simulink model "KAL_PID"  (R2019a)
settings: Solver=FixedStepAuto  StartTime=0.0  StopTime=4/speed  FixedStep=0.005  MaxStep=1e-2  MinStep=1e-3  RelTol=5e-3
PreLoadFcn:
  | helperSLCreateUtilityBus;
  | createCostmap;
StopFcn:
  | clear helperSLVisualizePath;
values from neighbouring files (symbols this model uses):
  costmap = vehicleCostmap(circuit, 'cellSize', res )    [createCostmap.m]    (also in helperSLVisualizePath.m = vehicleCostmap(costmapStruct.Costs,          'FreeThreshold')
  curvatures = zeros(561,1)    [createCostmap.m]
  refPoses = zeros(561, 3)    [createCostmap.m]
  speed = 0.1    [createCostmap.m]
  startPose = refPoses(1,:)    [createCostmap.m]
libraries: simulink_extras x3, simulink x2, autolibshared x1
settings Model: Creator=The MathWorks, Inc.  LastModifiedBy=mingz
settings SolverCC: ZeroCrossAlgorithm=Adaptive  DecoupledContinuousIntegration=on  MinimalZcImpactIntegration=on
settings DataIOCC: SaveFormat=Array  SaveOutput=off  SignalLogging=off  DSMLogging=off  SaveTime=off  ReturnWorkspaceOutputs=off
settings OptimizationCC: UseDivisionForNetSlopeComputation=on
settings DebuggingCC: PregeneratedLibrarySubsystemCodeDiagnostic=none  ArithmeticOperatorsInVariantConditions=warning
settings SFSimCC: SimUseLocalCustomCode=off
settings RTWCC: RTWUseLocalCustomCode=off

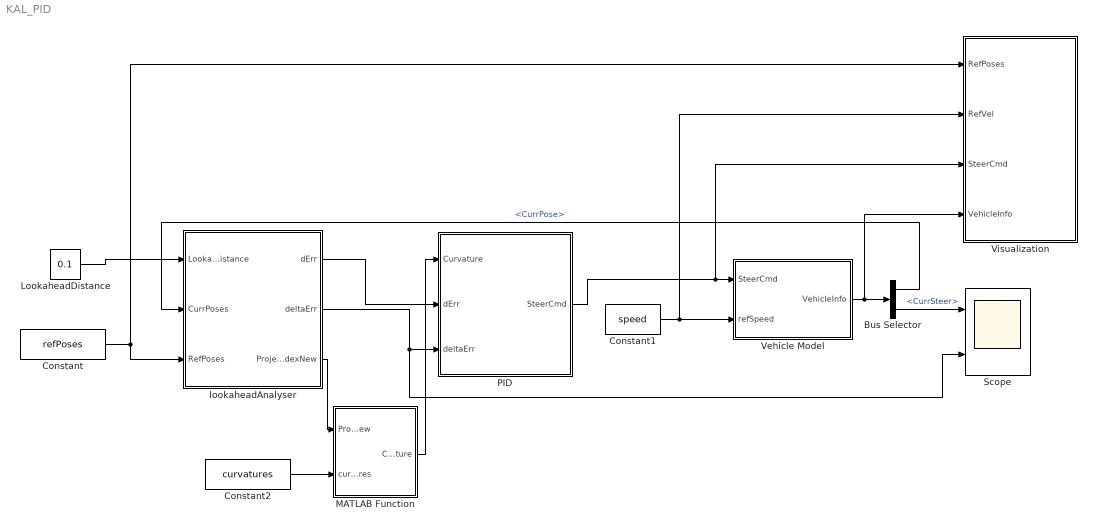
== system KAL_PID ==
  Bus Selector : BusSelector  OutputSignals=CurrPose,CurrSteer
  Constant : Constant  Value=refPoses
  Constant1 : Constant  Value=speed
  Constant2 : Constant  Value=curvatures
  LookaheadDistance : Constant  Value=0.1
  MATLAB Function : MATLAB Function  TreatAsAtomicUnit=on
  PID : Subsystem
  Scope : Scope  NumInputPorts=2
  Vehicle Model : Subsystem
  Visualization : Subsystem  mask{Costmap=costmap}
      mask prompts: Costmap "Vehicle costmap:"
      mask init:
      | validateattributes(Costmap, {'vehicleCostmap'}, {'scalar'});
      | 
      | varagout          = helperSLCreateUtilityStruct(Costmap);
      | vehicleDimsStruct = varagout{1};
      | costmapStruct     = varagout{2};
      mask DialogControl DescTextVar Prompt: Visualize simulation results.
  lookaheadAnalyser : Subsystem
  wires:
  Constant/1 -> Visualization/1(RefPoses), lookaheadAnalyser/3(RefPoses)
  Bus Selector/1 -> lookaheadAnalyser/2(CurrPoses)  "<CurrPose>"
  Bus Selector/2 -> Scope/1  "<CurrSteer>"
  Vehicle Model/1(VehicleInfo) -> Visualization/4(VehicleInfo), Bus Selector/1
  Constant1/1 -> Visualization/2(RefVel), Vehicle Model/2(refSpeed)
  lookaheadAnalyser/2(deltaErr) -> Scope/2, PID/3(deltaErr)
  lookaheadAnalyser/1(dErr) -> PID/2(dErr)
  lookaheadAnalyser/3(ProjectionLineIndexNew) -> MATLAB Function/1(ProjectionLineIndexNew)
  Constant2/1 -> MATLAB Function/2(curvatures)
  MATLAB Function/1(Curvature) -> PID/1(Curvature)
  PID/1(SteerCmd) -> Visualization/3(SteerCmd), Vehicle Model/1(SteerCmd)
  LookaheadDistance/1 -> lookaheadAnalyser/1(LookaheadDistance)

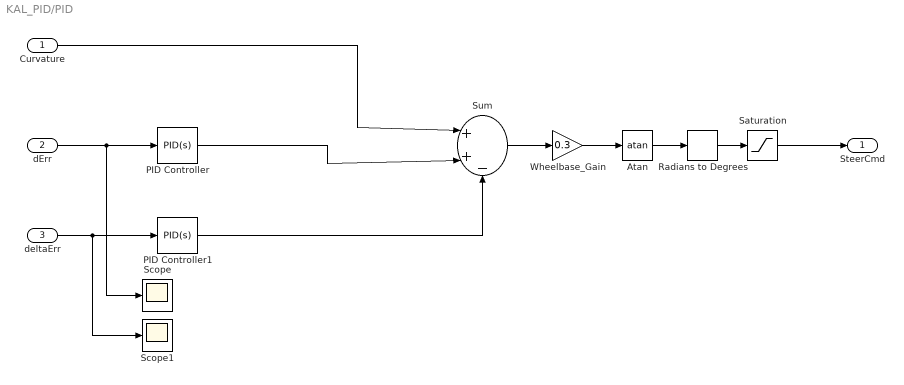
== system KAL_PID/PID ==
  Curvature : Inport
  dErr : Inport  Port=2
  deltaErr : Inport  Port=3
  Atan : Trigonometry  Operator=atan
  PID Controller : simulink/Continuous/PID Controller  Controller=PID  Form=Parallel  TimeDomain=Continuous-time  SampleTime=-1  IntegratorMethod=Forward Euler  FilterMethod=Forward Euler  ControllerParametersSource=internal  P=1  I=0  D=0.8  UseFilter=on  N=100  TunerSelectOption=Transfer Function Based (PID Tuner App)  InitialConditionSource=internal  InitialConditionForIntegrator=0  InitialConditionForFilter=0  DifferentiatorICPrevScaledInput=0  ExternalReset=none  TrackingMode=off  Kt=1  LimitOutput=off  UpperSaturationLimit=inf  LowerSaturationLimit=-inf  LinearizeAsGain=on  AntiWindupMode=none  Kb=1  POutMin=[]  POutMax=[]  IOutMin=[]  IOutMax=[]  DOutMin=[]  DOutMax=[]  NOutMin=[]  NOutMax=[]  SumOutMin=[]  SumOutMax=[]  SaturationOutMin=[]  SaturationOutMax=[]  PParamMin=[]  PParamMax=[]  IParamMin=[]  IParamMax=[]  DParamMin=[]  DParamMax=[]  NParamMin=[]  NParamMax=[]  KbParamMin=[]  KbParamMax=[]  KtParamMin=[]  KtParamMax=[]  KbOutMin=[]  KbOutMax=[]  KtOutMin=[]  KtOutMax=[]  IntegratorOutMin=[]  IntegratorOutMax=[]  FilterOutMin=[]  FilterOutMax=[]  SumI1OutMin=[]  SumI1OutMax=[]  SumI2OutMin=[]  SumI2OutMax=[]  SumI3OutMin=[]  SumI3OutMax=[]  SumI4OutMin=[]  SumI4OutMax=[]  SumDOutMin=[]  SumDOutMax=[]  DifferentiatorOutMin=[]  DifferentiatorOutMax=[]  FilterDiffOutCoefMin=[]  FilterDiffOutCoefMax=[]  ReciprocalOutMin=[]  ReciprocalOutMax=[]  SumDenOutMin=[]  SumDenOutMax=[]  SumNumOutMin=[]  SumNumOutMax=[]  DivideOutMin=[]  DivideOutMax=[]  IntegratorContinuousStateAttributes=''  IntegratorStateMustResolveToSignalObject=off  IntegratorRTWStateStorageClass=Auto  FilterContinuousStateAttributes=''  FilterStateMustResolveToSignalObject=off  FilterRTWStateStorageClass=Auto  ParallelPVariant=InternalParameters  IdealPVariant=Disabled  IVariant=InternalParameters  DVariant=InternalParameters  IntegratorVariant=Continuous  SatVariant=Disabled  AWVariant=Passthrough  PCopyVariant=Disabled  TRVariant=Disabled  FdbkBlocksVariant=Forward  IdealPFdbkVariant=Disabled  SatFdbkVariant=Disabled  DerivativeFilterVariant=ContFilter  NVariant=InternalParameters  NCopyVariant=Disabled  FilterICVariant=InternalICsFilter  IntegratorICVariant=InternalICs  ExternalResetVariant=Disabled  TRSumVariant=Passthrough  SumFdbkVariant=Disabled  SumVariant=Sum_PID
  PID Controller1 : simulink/Continuous/PID Controller  Controller=PID  Form=Parallel  TimeDomain=Continuous-time  SampleTime=-1  IntegratorMethod=Forward Euler  FilterMethod=Forward Euler  ControllerParametersSource=internal  P=2  I=0  D=0.6  UseFilter=on  N=100  TunerSelectOption=Transfer Function Based (PID Tuner App)  InitialConditionSource=internal  InitialConditionForIntegrator=0  InitialConditionForFilter=0  DifferentiatorICPrevScaledInput=0  ExternalReset=none  TrackingMode=off  Kt=1  LimitOutput=off  UpperSaturationLimit=inf  LowerSaturationLimit=-inf  LinearizeAsGain=on  AntiWindupMode=none  Kb=1  POutMin=[]  POutMax=[]  IOutMin=[]  IOutMax=[]  DOutMin=[]  DOutMax=[]  NOutMin=[]  NOutMax=[]  SumOutMin=[]  SumOutMax=[]  SaturationOutMin=[]  SaturationOutMax=[]  PParamMin=[]  PParamMax=[]  IParamMin=[]  IParamMax=[]  DParamMin=[]  DParamMax=[]  NParamMin=[]  NParamMax=[]  KbParamMin=[]  KbParamMax=[]  KtParamMin=[]  KtParamMax=[]  KbOutMin=[]  KbOutMax=[]  KtOutMin=[]  KtOutMax=[]  IntegratorOutMin=[]  IntegratorOutMax=[]  FilterOutMin=[]  FilterOutMax=[]  SumI1OutMin=[]  SumI1OutMax=[]  SumI2OutMin=[]  SumI2OutMax=[]  SumI3OutMin=[]  SumI3OutMax=[]  SumI4OutMin=[]  SumI4OutMax=[]  SumDOutMin=[]  SumDOutMax=[]  DifferentiatorOutMin=[]  DifferentiatorOutMax=[]  FilterDiffOutCoefMin=[]  FilterDiffOutCoefMax=[]  ReciprocalOutMin=[]  ReciprocalOutMax=[]  SumDenOutMin=[]  SumDenOutMax=[]  SumNumOutMin=[]  SumNumOutMax=[]  DivideOutMin=[]  DivideOutMax=[]  IntegratorContinuousStateAttributes=''  IntegratorStateMustResolveToSignalObject=off  IntegratorRTWStateStorageClass=Auto  FilterContinuousStateAttributes=''  FilterStateMustResolveToSignalObject=off  FilterRTWStateStorageClass=Auto  ParallelPVariant=InternalParameters  IdealPVariant=Disabled  IVariant=InternalParameters  DVariant=InternalParameters  IntegratorVariant=Continuous  SatVariant=Disabled  AWVariant=Passthrough  PCopyVariant=Disabled  TRVariant=Disabled  FdbkBlocksVariant=Forward  IdealPFdbkVariant=Disabled  SatFdbkVariant=Disabled  DerivativeFilterVariant=ContFilter  NVariant=InternalParameters  NCopyVariant=Disabled  FilterICVariant=InternalICsFilter  IntegratorICVariant=InternalICs  ExternalResetVariant=Disabled  TRSumVariant=Passthrough  SumFdbkVariant=Disabled  SumVariant=Sum_PID
  Radians to Degrees : simulink_extras/Transformations/Radians to Degrees
  Saturation : Saturate  UpperLimit=50  LowerLimit=-50
  Scope : Scope
  Scope1 : Scope
  Sum : Sum  Inputs=|++-
  Wheelbase_Gain : Gain  Gain=0.3
  SteerCmd : Outport
  wires:
  dErr/1 -> Scope/1, PID Controller/1
  PID Controller1/1 -> Sum/3
  Curvature/1 -> Sum/1
  Saturation/1 -> SteerCmd/1
  PID Controller/1 -> Sum/2
  Sum/1 -> Wheelbase_Gain/1
  Wheelbase_Gain/1 -> Atan/1
  Atan/1 -> Radians to Degrees/1
  Radians to Degrees/1 -> Saturation/1
  deltaErr/1 -> Scope1/1, PID Controller1/1

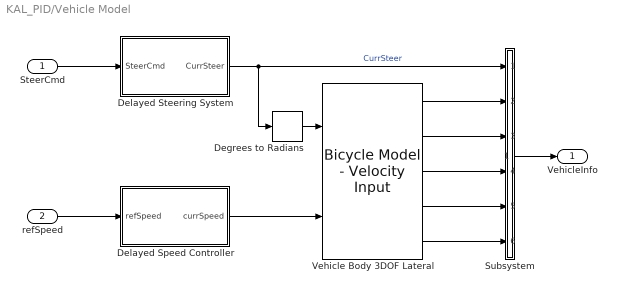
== system KAL_PID/Vehicle Model ==
  SteerCmd : Inport
  refSpeed : Inport  Port=2
  Degrees to Radians : simulink_extras/Transformations/Degrees to Radians
  Delayed Speed Controller : Subsystem
  Delayed Steering System : Subsystem
  Subsystem : Subsystem
  Vehicle Body 3DOF Lateral : autolibshared/Bicycle Model - Velocity Input  trackMode=Single (bicycle)  inputMode=External longitudinal forces  frontSteerMode=on  rearSteerMode=off  windMode=off  muMode=off  extFMode=off  extMMode=off  aMode=3  NF=2  NR=2  m=1.2  a=0.10  b=0.05  h=0.04  X_o=startPose(1)+cosd(startPose(3))*0.05  xdot_o=0  CalphaMode=off  sigmaMode=on  w=[1.4,1.4]  Cy_f=19e3  Cy_r=20e3  sigma_f=.1  sigma_r=.1  alpha_f_brk=[-.1 .1]  Cy_f_data=[-9e3 9e3]  alpha_r_brk=[-.1 .1]  Cy_r_data=[-9e3 9e3]  Y_o=startPose(2)+sind(startPose(3))*0.05  ydot_o=0  Izz=0.004  psi_o=deg2rad(startPose(3))  r_o=0  Af=2  Cd=.3  Cl=.1  Cpm=.1  beta_w=[0:0.01:0.3]  Cs=[0:0.03:0.9]  Cym=[0:0.01:0.3]  Pabs=101325  Tair=273  g=9.81  mu=1  xdot_tol=0.01  Fznom=5000  Fxtire_sat=1e6  Fytire_sat=1e6  longOff=0  latOff=0  vertOff=0
      settings: SourceProductName=Powertrain Blockset  SourceProductBaseCode=PW
  VehicleInfo : Outport
  wires:
  Delayed Speed Controller/1(currSpeed) -> Vehicle Body 3DOF Lateral/2
  Degrees to Radians/1 -> Vehicle Body 3DOF Lateral/1
  Delayed Steering System/1(CurrSteer) -> Degrees to Radians/1, Subsystem/1(CurrSteer)  "CurrSteer"
  SteerCmd/1 -> Delayed Steering System/1(SteerCmd)
  Subsystem/1(VehicleInfo) -> VehicleInfo/1
  Vehicle Body 3DOF Lateral/1 -> Subsystem/2(Info)
  Vehicle Body 3DOF Lateral/2 -> Subsystem/3(In3)
  Vehicle Body 3DOF Lateral/3 -> Subsystem/4(In4)
  Vehicle Body 3DOF Lateral/4 -> Subsystem/5(In6)
  Vehicle Body 3DOF Lateral/5 -> Subsystem/6(<Direction>)
  refSpeed/1 -> Delayed Speed Controller/1(refSpeed)

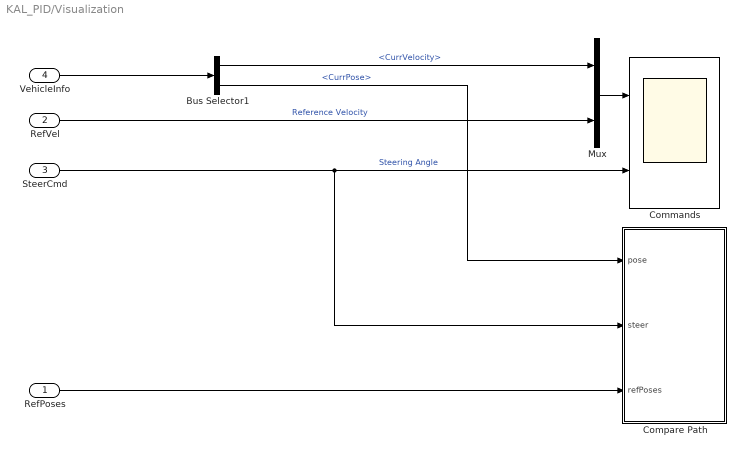
== system KAL_PID/Visualization ==
  RefPoses : Inport
  RefVel : Inport  Port=2
  SteerCmd : Inport  Port=3
  VehicleInfo : Inport  Port=4
  Bus Selector1 : BusSelector  OutputSignals=CurrVelocity,CurrPose
  Commands : Scope  NumInputPorts=2
  Compare Path : MATLAB Function  TreatAsAtomicUnit=on
  Mux : Mux  Inputs=2
  wires:
  Bus Selector1/1 -> Mux/1  "<CurrVelocity>"
  Bus Selector1/2 -> Compare Path/1(pose)  "<CurrPose>"
  RefVel/1 -> Mux/2  "Reference Velocity"
  Mux/1 -> Commands/1
  SteerCmd/1 -> Compare Path/2(steer), Commands/2  "Steering Angle"
  VehicleInfo/1 -> Bus Selector1/1
  RefPoses/1 -> Compare Path/3(refPoses)

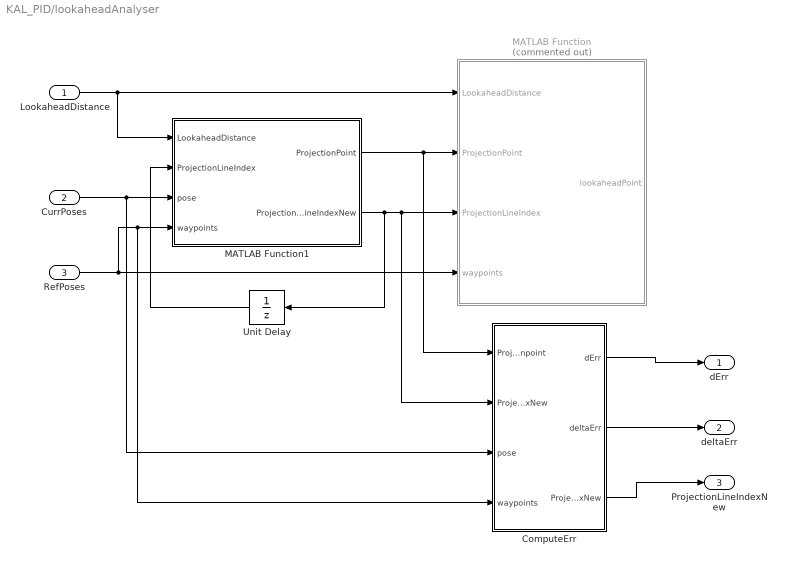
== system KAL_PID/lookaheadAnalyser ==
  LookaheadDistance : Inport
  CurrPoses : Inport  Port=2
  RefPoses : Inport  Port=3
  ComputeErr : MATLAB Function  TreatAsAtomicUnit=on
  MATLAB Function : MATLAB Function  Commented=on  TreatAsAtomicUnit=on
  MATLAB Function1 : MATLAB Function  TreatAsAtomicUnit=on
  Unit Delay : UnitDelay  SampleTime=-1  HasFrameUpgradeWarning=on
  dErr : Outport
  deltaErr : Outport  Port=2
  ProjectionLineIndexNew : Outport  Port=3
  wires:
  LookaheadDistance/1 -> MATLAB Function1/1(LookaheadDistance), MATLAB Function/1(LookaheadDistance)
  CurrPoses/1 -> ComputeErr/3(pose), MATLAB Function1/3(pose)
  Unit Delay/1 -> MATLAB Function1/2(ProjectionLineIndex)
  RefPoses/1 -> ComputeErr/4(waypoints), MATLAB Function1/4(waypoints), MATLAB Function/4(waypoints)
  MATLAB Function1/2(ProjectionLineIndexNew) -> Unit Delay/1, ComputeErr/2("ProjectionLineIndexNew "), MATLAB Function/3(ProjectionLineIndex)
  MATLAB Function1/1(ProjectionPoint) -> ComputeErr/1(Projectionpoint), MATLAB Function/2(ProjectionPoint)
  ComputeErr/1(dErr) -> dErr/1
  ComputeErr/2(deltaErr) -> deltaErr/1
  ComputeErr/3(ProjectionLineIndexNew) -> ProjectionLineIndexNew/1

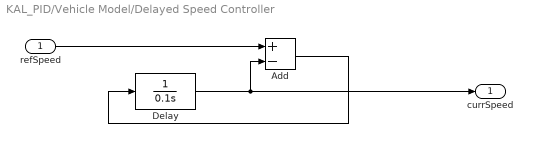
== system KAL_PID/Vehicle Model/Delayed Speed Controller ==
  refSpeed : Inport
  Add : Sum  Inputs=+-
  Delay : TransferFcn  Denominator=[0.1 0]
  currSpeed : Outport
  wires:
  Add/1 -> Delay/1
  refSpeed/1 -> Add/1
  Delay/1 -> currSpeed/1, Add/2

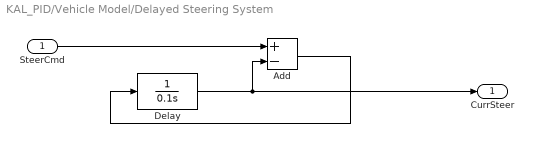
== system KAL_PID/Vehicle Model/Delayed Steering System ==
  SteerCmd : Inport
  Add : Sum  Inputs=+-
  Delay : TransferFcn  Denominator=[0.1 0]
  CurrSteer : Outport
  wires:
  Add/1 -> Delay/1
  SteerCmd/1 -> Add/1
  Delay/1 -> CurrSteer/1, Add/2

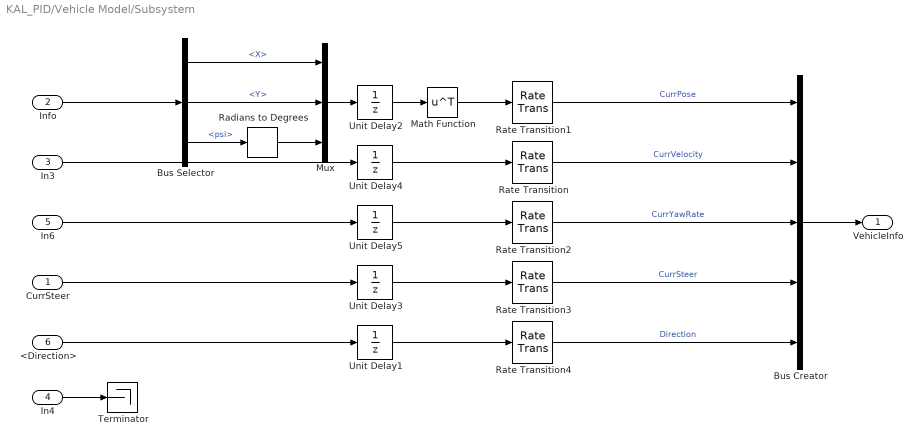
== system KAL_PID/Vehicle Model/Subsystem ==
  CurrSteer : Inport
  Info : Inport  Port=2
  In3 : Inport  Port=3
  In4 : Inport  Port=4
  In6 : Inport  Port=5
  <Direction> : Inport  Port=6
  Bus Creator : BusCreator  Inputs=5  OutDataTypeStr=Bus: vehicleInfoBus  NonVirtualBus=on
  Bus Selector : BusSelector  OutputSignals=InertFrm.RearAxl.Disp.X,InertFrm.RearAxl.Disp.Y,InertFrm.Cg.Ang.psi
  Math Function : Math  Operator=transpose  SaturateOnIntegerOverflow=on
  Mux : Mux  Inputs=3
  Radians to Degrees : simulink_extras/Transformations/Radians to Degrees
  Rate Transition : RateTransition  OutPortSampleTime=0.1
  Rate Transition1 : RateTransition  InitialCondition=startPose  OutPortSampleTime=0.1
  Rate Transition2 : RateTransition  OutPortSampleTime=0.1
  Rate Transition3 : RateTransition  OutPortSampleTime=0.1
  Rate Transition4 : RateTransition  InitialCondition=1  OutPortSampleTime=0.1
  Terminator : Terminator
  Unit Delay1 : UnitDelay  InitialCondition=1  SampleTime=-1  HasFrameUpgradeWarning=on
  Unit Delay2 : UnitDelay  InitialCondition=startPose  SampleTime=-1  HasFrameUpgradeWarning=on
  Unit Delay3 : UnitDelay  SampleTime=-1  HasFrameUpgradeWarning=on
  Unit Delay4 : UnitDelay  SampleTime=-1  HasFrameUpgradeWarning=on
  Unit Delay5 : UnitDelay  SampleTime=-1  HasFrameUpgradeWarning=on
  VehicleInfo : Outport
  wires:
  Unit Delay1/1 -> Rate Transition4/1
  CurrSteer/1 -> Unit Delay3/1
  Unit Delay5/1 -> Rate Transition2/1
  <Direction>/1 -> Unit Delay1/1
  Unit Delay4/1 -> Rate Transition/1
  Math Function/1 -> Rate Transition1/1
  Rate Transition/1 -> Bus Creator/2  "CurrVelocity"
  Unit Delay3/1 -> Rate Transition3/1
  Rate Transition3/1 -> Bus Creator/4  "CurrSteer"
  Rate Transition1/1 -> Bus Creator/1  "CurrPose"
  Rate Transition2/1 -> Bus Creator/3  "CurrYawRate"
  Rate Transition4/1 -> Bus Creator/5  "Direction"
  Unit Delay2/1 -> Math Function/1
  Info/1 -> Bus Selector/1
  Radians to Degrees/1 -> Mux/3
  Bus Selector/2 -> Mux/2  "<Y>"
  Bus Selector/1 -> Mux/1  "<X>"
  Mux/1 -> Unit Delay2/1
  In3/1 -> Unit Delay4/1
  In4/1 -> Terminator/1
  In6/1 -> Unit Delay5/1
  Bus Selector/3 -> Radians to Degrees/1  "<psi>"
  Bus Creator/1 -> VehicleInfo/1

== matlab function KAL_PID/lookaheadAnalyser/MATLAB Function ==
  data: LookaheadDistance input; lookaheadPoint output; ProjectionPoint input; ProjectionLineIndex input; waypoints input
function lookaheadPoint = getLookaheadPoint(LookaheadDistance, ProjectionPoint, ProjectionLineIndex, waypoints)
    %getLookaheadPoint Find the look ahead point on the path past
    %the Projection point.

    if size(waypoints, 1) == 1
        lookaheadPoint = waypoints(1,1:2);
        return;
    end

    % First check the current line segment
    dist = norm(ProjectionPoint-waypoints(ProjectionLineIndex+1,1:2));
    lookaheadStartPt = ProjectionPoint;
    lookaheadEndPt = waypoints(ProjectionLineIndex+1,1:2);
    overshootDist = dist - LookaheadDistance;
    lookaheadIdx = ProjectionLineIndex;

    % If the remaining path on current line segment is not long
    % enough for look ahead, check the waypoints past current line
    % segment.
    while overshootDist < 0 && lookaheadIdx < size(waypoints,1)-1
        lookaheadIdx = lookaheadIdx + 1;

        lookaheadStartPt = waypoints(lookaheadIdx,1:2);
        lookaheadEndPt = waypoints(lookaheadIdx+1,1:2);
        dist = dist + norm(lookaheadStartPt-lookaheadEndPt);

        overshootDist = dist - LookaheadDistance;
    end

    % Find the exact look ahead point by interpolating between the
    % start and end point of the line segment on which the
    % lookahead point lies.
    alpha = overshootDist/norm(lookaheadStartPt - lookaheadEndPt);
    if alpha > 0
        lookaheadPoint = (alpha.*lookaheadStartPt + (1-alpha).*lookaheadEndPt)';
    else
        lookaheadPoint = lookaheadEndPt';
    end
end

== matlab function KAL_PID/lookaheadAnalyser/ComputeErr ==
  data: Projectionpoint input; dErr output; ProjectionLineIndexNew input; pose input; waypoints input; deltaErr output; ProjectionLineIndexNew output
function [dErr,deltaErr,ProjectionLineIndexNew]    = computErr(Projectionpoint, ProjectionLineIndexNew,pose,waypoints)
pose = reshape(pose,1,3);

dErr = norm(Projectionpoint(1:2) - pose(1:2));
delta = atan2(waypoints(ProjectionLineIndexNew+1,2) - Projectionpoint(1,2), waypoints(ProjectionLineIndexNew+1,1) - Projectionpoint(1,1));
if delta<0
    delta = delta+2*pi;
end
deltaErr = pose(3)- delta*180/pi;
return;
end

== matlab function KAL_PID/lookaheadAnalyser/MATLAB Function1 ==
  data: LookaheadDistance input; ProjectionPoint output; ProjectionLineIndex input; pose input; waypoints input; ProjectionLineIndexNew output
function [ProjectionPoint, ProjectionLineIndexNew] = computeProjectionPoint(LookaheadDistance, ProjectionLineIndex, pose, waypoints)
    %computeProjectionPoint Find closest point past the last Projection point
    
    pose = reshape(pose,1,3);
    searchFlag = false;
    % If Projection point is not initialized, start searching from
    % first waypoint
    if ProjectionLineIndex == 0
        searchFlag = true;
        % ProjectionPoint = waypoints(1,1:2);
        ProjectionLineIndexNew = cast(1, 'like', pose);
    else
        ProjectionLineIndexNew = ProjectionLineIndex;
    end

    if size(waypoints, 1) == 1
        ProjectionPoint = waypoints(1,1:2);
        return;
    end
    % Start searching from the current projection line segment
    [ProjectionPoint, minDistance] = ...
        closestPointOnLine(waypoints(ProjectionLineIndexNew,1:2), ...
        waypoints(ProjectionLineIndexNew+1,1:2), pose(1:2));

    dist = norm(ProjectionPoint - waypoints(ProjectionLineIndexNew+1,1:2));
    %dErr = norm(ProjectionPoint(1:2) - pose(1:2));
    %delta = atan2(ProjectionPoint(1,2)- waypoints(ProjectionLineIndexNew+1,2), ProjectionPoint(1,1)-waypoints(ProjectionLineIndexNew+1,1));
    %deltaErr = delta - pose(3)*pi/180;
    for i = ProjectionLineIndexNew+1:size(waypoints,1)-1

        if ~searchFlag && dist > LookaheadDistance
            break;
        end
        dist = dist + norm(waypoints(i,1:2) - waypoints(i+1,1:2));
        % Check the remaining waypoints
        [tempPoint, tempDistance] = ...
            closestPointOnLine(waypoints(i,1:2), ...
            waypoints(i+1,1:2), pose(1:2));
        %delta = atan2(ProjectionPoint(1,2)-(waypoints(i+1,2))/(ProjectionPoint(1,1)-waypoints(i+1,1)));
        if tempDistance < minDistance
            minDistance = tempDistance;
            ProjectionPoint = tempPoint;
            ProjectionLineIndexNew = cast(i, 'like', pose);
        end
    end
end

== matlab function KAL_PID/MATLAB Function ==
  data: ProjectionLineIndexNew input; Curvature output; curvatures input
function Curvature  = computErr(ProjectionLineIndexNew,curvatures)
double curvatureidx;
curvatureidx = ProjectionLineIndexNew+10;
if curvatureidx > 561
    curvatureidx = 561;
end
Curvature = curvatures(curvatureidx);
return
end

== matlab function KAL_PID/Visualization/Compare Path ==
  settings: updateMethod=DISCRETE  sampleTime=0.1
  data: pose input size=[1 3]; steer input; refPoses input; costmapStruct parameter; vehicleDimsStruct parameter
function visualizePath(pose, steer, refPoses, costmapStruct, vehicleDimsStruct)

%visualizePath Display simulation results.

coder.extrinsic('helperSLVisualizePath');

helperSLVisualizePath(pose, steer, refPoses, costmapStruct, vehicleDimsStruct)
